simulink model "product_mix_1"  (R2017b)
settings: Solver=FixedStepDiscrete  StartTime=0.0  StopTime=10.0  FixedStep=0.200000  RelTol=1e-3
settings Model: Creator=hbourbou  LastModifiedBy=hbourbou
settings DataIOCC: SaveFormat=StructureWithTime
settings OptimizationCC: LifeSpan=inf
settings DebuggingCC: SFExecutionAtInitializationDiag=none
settings HardwareCC: ProdBitPerSizeT=32  ProdBitPerPtrDiffT=32  ProdWordSize=32  ProdHWDeviceType=Specified
settings CodeAppCC: StateflowObjectComments=on

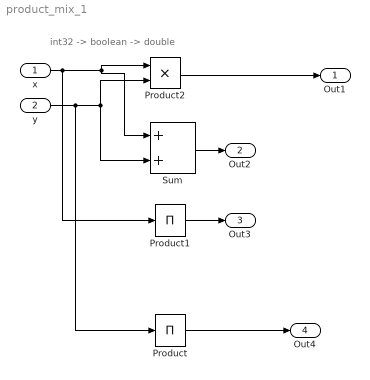
== system product_mix_1 ==
  note: int32 -> boolean -> double
  x : Inport  OutDataTypeStr=uint8  PortDimensions=3
  y : Inport  Port=2  OutDataTypeStr=uint16
  Product : Product  Inputs=1
  Product1 : Product  Inputs=*
  Product2 : Product  Inputs=**
  Sum : Sum  Inputs=2
  Out1 : Outport
  Out2 : Outport  Port=2
  Out3 : Outport  Port=3
  Out4 : Outport  Port=4
  wires:
  Product2/1 -> Out1/1
  y/1 -> Product/1, Product2/2, Sum/2
  Sum/1 -> Out2/1
  x/1 -> Product1/1, Sum/1, Product2/1
  Product1/1 -> Out3/1
  Product/1 -> Out4/1
